simulink model "proposed_1"  (R2021b)
settings: Solver=VariableStepAuto  StartTime=0.0  StopTime=0.7  RelTol=1e-3
values from neighbouring files (symbols this model uses):
  Ts_Control = 1e-05    [final.mat]    (also in reykt.mat = 2.6455026455e-05)
libraries: fl_lib x25, nesl_utility x22, ee_lib x11, spsPWMGeneratorDCDCLib x10, slpidlib x7, eeGeneralControl x3, spsPLLLib x1, spsAlphaBetaZerotodq0Lib x1, spsDiscreteVariableTimeDelayLib x1
(part 2 of 2)

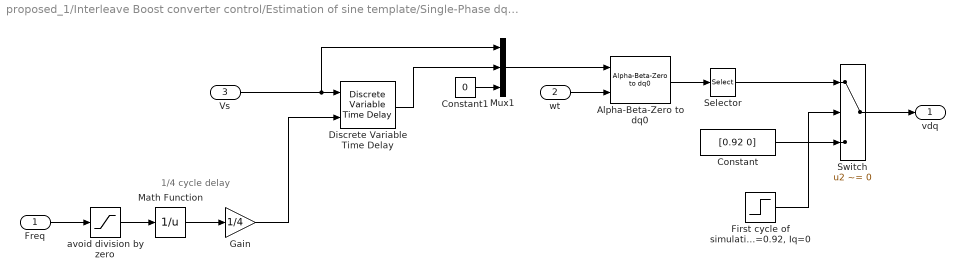
== system proposed_1/Interleave Boost converter control/Estimation of sine template/Single-Phase dq Transform ==
  note: 1/4 cycle delay
  Freq : Inport
  wt : Inport  Port=2
  Vs : Inport  Port=3
  Alpha-Beta-Zero to dq0 : spsAlphaBetaZerotodq0Lib/Alpha-Beta-Zero to dq0  Alignment=90 degrees behind phase A axis
      settings: SourceProductBaseCode=PS
  Constant : Constant  Value=[0.92 0]
  Constant1 : Constant  Value=0
  Discrete Variable Time Delay : spsDiscreteVariableTimeDelayLib/Discrete Variable Time Delay  MaxDelay=1  InitialValue=0  Ts=Ts_Control  DFT=on
      settings: SourceProductBaseCode=PS
  "First cycle of simulation Id=0.92, Iq=0" : Step  Time=1/50  SampleTime=Ts_Control
  Gain : Gain  Gain=1/4
  Math Function : Math  Operator=reciprocal  SignedPower=on  SaturateOnIntegerOverflow=on
  Mux1 : Mux  Inputs=3
  Selector : Selector  InputPortWidth=3  IndexOptions=Index vector (dialog)  Indices=[1 2]  OutputSizes=1
  Switch : Switch  Criteria=u2 ~= 0
  avoid division by zero : Saturate  UpperLimit=70  LowerLimit=40
  vdq : Outport  VectorParamsAs1DForOutWhenUnconnected=off
  wires:
  Constant1/1 -> Mux1/3
  Discrete Variable Time Delay/1 -> Mux1/2
  Mux1/1 -> Alpha-Beta-Zero to dq0/1
  Vs/1 -> Discrete Variable Time Delay/1, Mux1/1
  wt/1 -> Alpha-Beta-Zero to dq0/2
  Alpha-Beta-Zero to dq0/1 -> Selector/1
  Freq/1 -> avoid division by zero/1
  avoid division by zero/1 -> Math Function/1
  Math Function/1 -> Gain/1
  Gain/1 -> Discrete Variable Time Delay/2
  Selector/1 -> Switch/1
  Switch/1 -> vdq/1
  Constant/1 -> Switch/3
  "First cycle of simulation Id=0.92, Iq=0"/1 -> Switch/2

== matlab function proposed_1/Interleave Boost converter control/Estimation of sine template/MATLAB Function ==
  data: vd input; us output; vq input; wt input
function us = fcn(vd, vq, wt)
Vm=sqrt(vd^2+vq^2);
Vd=Vm*sin(wt);
us = Vd/Vm;
